simulink model "vehicle_cmd"  (R2018b)
settings: Solver=VariableStepAuto  StartTime=0.0  StopTime=inf  RelTol=1e-3
undefined symbols (not defined in the file): AccelCmd, BrakeCmd, CtrlCmd, TwistCmd
libraries: simulink x5, robotlib x3
settings Model: Creator=phuris  LastModifiedBy=phuris

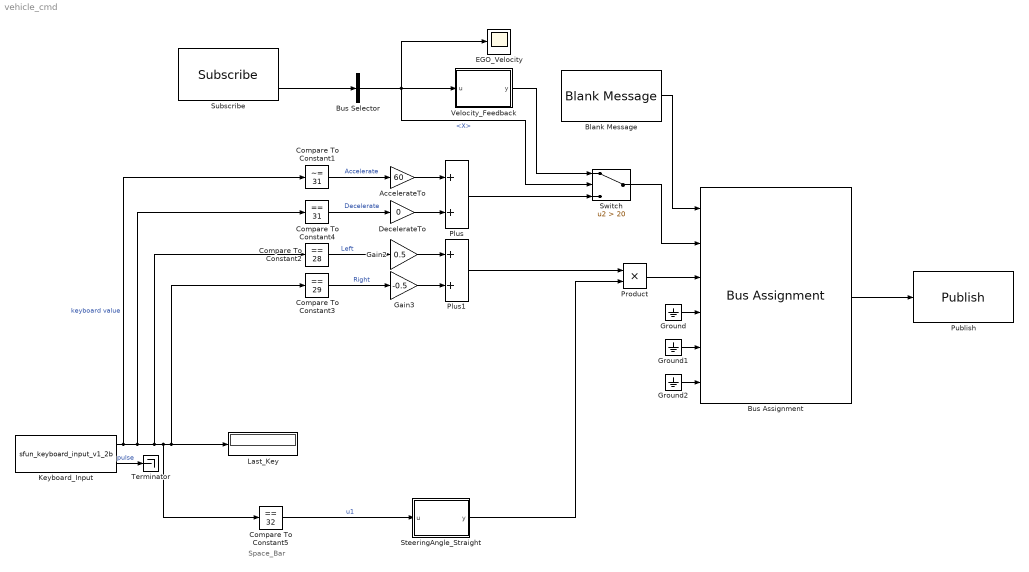
== system vehicle_cmd ==
  note: Space_Bar
  AccelerateTo : Gain  Gain=60  OutDataTypeStr=double
  Blank Message : robotlib/Blank Message  messageClass=Message  entityType=autoware_msgs/VehicleCmd  messageType=autoware_msgs/VehicleCmd  SampleTime=inf
      settings: SourceProductBaseCode=RO
  Bus Assignment : BusAssignment  AssignedSignals=TwistCmd.Twist.Linear.X,TwistCmd.Twist.Angular.Z,AccelCmd.Accel,CtrlCmd.LinearAcceleration,BrakeCmd.Brake
  Bus Selector : BusSelector  OutputSignals=Twist.Linear.X
  Compare To Constant1 : simulink/Logic and Bit Operations/Compare To Constant  relop=~=  const=31  OutDataTypeStr=boolean
  Compare To Constant2 : simulink/Logic and Bit Operations/Compare To Constant  relop===  const=28  OutDataTypeStr=boolean
  Compare To Constant3 : simulink/Logic and Bit Operations/Compare To Constant  relop===  const=29  OutDataTypeStr=boolean
  Compare To Constant4 : simulink/Logic and Bit Operations/Compare To Constant  relop===  const=31  OutDataTypeStr=boolean
  Compare To Constant5 : simulink/Logic and Bit Operations/Compare To Constant  relop===  const=32  OutDataTypeStr=boolean
  DecelerateTo : Gain  Gain=0  ParamDataTypeStr=double  OutDataTypeStr=double
  EGO_Velocity : Scope
  Gain2 : Gain  Gain=0.5  OutDataTypeStr=double
  Gain3 : Gain  Gain=-0.5  OutDataTypeStr=double
  Ground : Ground
  Ground1 : Ground
  Ground2 : Ground
  Keyboard_Input : M-S-Function  FunctionName=sfun_keyboard_input_v1_2b  mask(Keyboard Input){}
      mask help: Keyboard Input
      mask Display: fprintf('Keyboard');
  Last_Key : Display
  Plus : Sum
  Plus1 : Sum
  Product : Product
  Publish : robotlib/Publish  topicSource=Select from ROS network  topic=/vehicle_cmd  messageType=autoware_msgs/VehicleCmd  messageQueueLength=1
      settings: SourceProductBaseCode=RO
  SteeringAngle_Straight : MATLAB Function  TreatAsAtomicUnit=on
  Subscribe : robotlib/Subscribe  topicSource=Select from ROS network  topic=/sim_velocity  messageType=geometry_msgs/TwistStamped  sampleTime=-1  messageQueueLength=1
      settings: SourceProductBaseCode=RO
  Switch : Switch  Criteria=u2 > Threshold  Threshold=20
  Terminator : Terminator
  Velocity_Feedback : MATLAB Function  TreatAsAtomicUnit=on
  wires:
  Blank Message/1 -> Bus Assignment/1
  Bus Assignment/1 -> Publish/1
  Plus1/1 -> Product/1
  Keyboard_Input/1 -> Compare To Constant2/1, Compare To Constant5/1, Compare To Constant3/1, Last_Key/1, Compare To Constant4/1, Compare To Constant1/1  "keyboard value"
  Compare To Constant4/1 -> DecelerateTo/1  "Decelerate"
  Compare To Constant1/1 -> AccelerateTo/1  "Accelerate"
  AccelerateTo/1 -> Plus/1
  DecelerateTo/1 -> Plus/2
  Plus/1 -> Switch/3
  Compare To Constant2/1 -> Gain2/1  "Left"
  Compare To Constant3/1 -> Gain3/1  "Right"
  Gain2/1 -> Plus1/1
  Gain3/1 -> Plus1/2
  Compare To Constant5/1 -> SteeringAngle_Straight/1(u)  "u1"
  SteeringAngle_Straight/1(y) -> Product/2
  Product/1 -> Bus Assignment/3
  Subscribe/2 -> Bus Selector/1
  Bus Selector/1 -> EGO_Velocity/1, Switch/2, Velocity_Feedback/1(u)  "<X>"
  Velocity_Feedback/1(y) -> Switch/1
  Switch/1 -> Bus Assignment/2
  Ground/1 -> Bus Assignment/4
  Ground1/1 -> Bus Assignment/5
  Ground2/1 -> Bus Assignment/6
  Keyboard_Input/2 -> Terminator/1  "pulse"

== matlab function vehicle_cmd/Velocity_Feedback ==
  data: u input; y output
function y = fcn(u)
    if u > 20
        y = 20;
    else
        y = u;
    end

== matlab function vehicle_cmd/SteeringAngle_Straight ==
  data: u input; y output
function y = fcn(u)
    if u == 1
        y = 0;
    else 
        y = 1;
    end
